simulink model "simulink7_4yanz"  (R2017a)
settings: Solver=VariableStepAuto  StartTime=0.0  StopTime=10.0  RelTol=1e-3
settings Model: Creator=adi  LastModifiedBy=adi

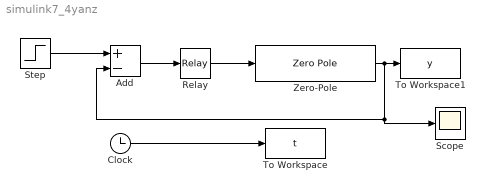
== system simulink7_4yanz ==
  Add : Sum  Inputs=+-
  Clock : Clock
      settings: Decimation=30
  Relay : Relay  OnSwitchValue=0  OffSwitchValue=0  OffOutputValue=-1
  Scope : Scope
  Step : Step  Time=0  SampleTime=0
  To Workspace : ToWorkspace  VariableName=t  SampleTime=-1
  To Workspace1 : ToWorkspace  VariableName=y  SampleTime=-1
  Zero-Pole : ZeroPole  Zeros=[]  Poles=[0 -3 -2]  Gain=8
  wires:
  Zero-Pole/1 -> Scope/1, Add/2, To Workspace1/1
  Clock/1 -> To Workspace/1
  Add/1 -> Relay/1
  Relay/1 -> Zero-Pole/1
  Step/1 -> Add/1
